simulink model "DriverInLoopSpeedgoat"  (R2021a)
settings: Solver=ode3  StartTime=0.0  StopTime=30  FixedStep=1e-3  RelTol=5e-3  EnableMultiTasking=on
StartFcn:
  | % tic
  | % tg2.start;
StopFcn:
  | % tg2.stop;
  | % toc
model workspace (MAT data in the model file):
  A_mu = 10
  B_reff = 8.386
  Cz = 7766.25
  DCT_Param.Transmission.Ratios = [3.78 2.18 1.43 1.03 0.935 0.84]
  DCT_Param.Transmission.Shaft_Inertia_Odd = 0.0023
  DCT_Param.Transmission.Shaft_Inertia_Even = 0.0009
  DCT_Param.Transmission.Shaft_Inertia_Output = 0.008
  DCT_Param.Transmission.Gear_Inertia = 0.001
  DCT_Param.Transmission.Gear_Efficiency = 0.94
  DCT_Param.Transmission.Gear_Ang_Vel_Thr = 0.01
  DCT_Param.Transmission.Shaft_Velocity_Odd = 0
  DCT_Param.Transmission.Shaft_Velocity_Even = 0
  DCT_Param.Transmission.Shaft_Velocity_Output = 0
  DCT_Param.Transmission.Gear_Initial_Velocity = 0
  DCT_Param.Transmission.Abstract.Compliance = 100000
  DCT_Param.Transmission.Abstract.Damping = 10000
  DCT_Param.Transmission.Abstract.Ratio_Time_Const = 0.05
  DCT_Param.Transmission.Abstract.Shift_Gear_Delay = 25
  DCT_Param.Clutch.Torque_Radius = 130
  DCT_Param.Clutch.Num_Friction_Surfaces = 4
  DCT_Param.Clutch.Engagement_Piston_Area = 0.001
  DCT_Param.Clutch.Kinetic_Friction_Coeff = 0.3
  DCT_Param.Clutch.Static_Friction_Coeff = 0.31
  DCT_Param.Clutch.Derating_Factor = 1
  DCT_Param.Clutch.Clutch_Velocity_Tolerance = 0.001
  DCT_Param.Clutch.Threshold_Pressure = 1
  DCT_Param.Clutch.Drag_Torque_Coeff = 0
  DCT_Param.Dog_Clutch.Max_Torque = 1000
  DCT_Param.Dog_Clutch.Teeth_Mean_Radius = 50
  DCT_Param.Dog_Clutch.Tooth_Height = 10
  DCT_Param.Dog_Clutch.Ring_Hub_Clearance = 3
  DCT_Param.Dog_Clutch.Ring_Stop_Stiffness = 1000000
  DCT_Param.Dog_Clutch.Ring_Stop_Damping = 1000
  DCT_Param.Dog_Clutch.Shift_Linkage_Damping = 100
  DCT_Param.Dog_Clutch.Max_Engage_Velocity = 1000000
  DCT_Param.Dog_Clutch.Tooth_Engage_Overlap = 3
  DCT_Param.Vehicle.Mass = 1600
  DCT_Param.Vehicle.Wheels_Per_Axle = 2
  DCT_Param.Vehicle.Distance_CG_FrontAxle = 1.7
  DCT_Param.Vehicle.Distance_CG_RearAxle = 2
  DCT_Param.Vehicle.Distance_CG_Ground = 0.5
  DCT_Param.Vehicle.Frontal_Area = 3
  DCT_Param.Vehicle.Aero_Drag_Coeff = 0.4
  DCT_Param.Vehicle.Initial_Velocity = 0
  DCT_Param.Vehicle.Final_Drive_Ratio = 3.7
  DCT_Param.Vehicle.Final_Drive_Efficiency = 0.86
  DCT_Param.Vehicle.Final_Drive_Vel_Thresh = 0.01
  DCT_Param.Vehicle.Side_Shaft_Inertia = 0.01
  DCT_Param.Vehicle.Side_Shaft_Initial_Velocity = 0
  DCT_Param.Vehicle.Tire.Radius = 0.312
  DCT_Param.Vehicle.Tire.Inertia = 0.5
  DCT_Param.Vehicle.Tire.Initial_Velocity = 0
  DCT_Param.Vehicle.Tire.Slip_Vel_Thresh = 0.1
  DCT_Param.Vehicle.Tire.Nominal_Vertical_Load = 4000
  DCT_Param.Vehicle.Tire.C_Coeff = 1.685
  DCT_Param.Vehicle.Tire.D_Coeff = [1.21 -0.037]
  DCT_Param.Vehicle.Tire.E_Coeff = [0.344 0.095 -0.02 0]
  DCT_Param.Vehicle.Tire.BCD_Coeff = [21.51 -0.163 0.245]
  DCT_Param.Vehicle.Tire.H_Coeff = [-0.002 0.002]
  DCT_Param.Vehicle.Tire.V_Coeff = [0 0]
  DCT_Param.ICE.Max_Power = 100000
  DCT_Param.ICE.Speed_At_Max_Power = 5500
  DCT_Param.ICE.Max_Speed = 7000
  DCT_Param.ICE.Stall_Speed = 200
  DCT_Param.ICE.Shaft_Inertia = 0.2
  DCT_Param.ICE.Initial_Velocity = 800
  DCT_Param.ICE.Idle_Ref_Spd = 800
  DCT_Param.ICE.Engine_Time_Constant = 0.2
  DCT_Param.ICE.Initial_Normalized_Throttle = 0
  DCT_Param.ICE.Speed_Threshold = 20
  DCT_Param.ICE.FC.Speed_Vector = [0 368.421052632 736.842105263 1105.26315789 1473.68421053 1842.10526316 2210.52631579 2578.94736842 2947.36842105 3315.78947368 3684.21052632 4052.63157895 4421.05263158 4789.47368421 5157.89473684 5526.31578947 5894.73684211 6263.15789474 6631.57894737 7000]
  DCT_Param.ICE.FC.Torque_Vector = [0 10.5263157895 21.0526315789 31.5789473684 42.1052631579 52.6315789474 63.1578947368 73.6842105263 84.2105263158 94.7368421053 105.263157895 115.789473684 126.315789474 136.842105263 147.368421053 157.894736842 168.421052632 178.947368421 189.473684211 200]
  DCT_Param.ICE.FC.Consumption_Table = [0.262945178015 0.225304787522 0.201465019624 0.191425874321 0.195187351614 0.212749451502 0.244112173984 0.289275519063 0.348239486736 0.421004077004 0.507569289868 0.607935125326 ... (400 elements, 20x20)]
  DCT_Param.Shift_Map_Example.Pedal_Positions = [0.1 0.4 0.5 0.9]
  DCT_Param.Shift_Map_Example.Upshift_Speeds = [11  20  26  34.5  43; 14  26  35  44.5  55; 17  31  42  52.5  65; 21  39  52  66.5  80]
  DCT_Param.Shift_Map_Example.Downshift_Speeds = [8.9  17  23.6  32.4  40.8; 11.5  22.7  32  41.6  52.2; 14  27  38.1  50  62; 18  33  48  62.6  76.2]
  DCT_Param.Shift_Map_ORIG.Pedal_Positions = [0.1 0.4 0.5 0.9]
  DCT_Param.Shift_Map_ORIG.Upshift_Speeds = [11.5  23.5  35.5  45.5  55.5; 14.5  26.5  38.5  48.5  58.5; 17.5  29.5  41.5  51.5  61.5; 20.5  32.5  44.5  54.5  64.5]
  DCT_Param.Shift_Map_ORIG.Downshift_Speeds = [8.5  20.5  32.5  42.5  52.5; 11.5  23.5  35.5  45.5  55.5; 14.5  26.5  38.5  48.5  58.5; 17.5  29.5  41.5  51.5  61.5]
  DCT_Param.Shift_Map_OPT.Pedal_Positions = [0.1 0.4 0.5 0.9]
  DCT_Param.Shift_Map_OPT.Upshift_Speeds = [17.8469  29.8469  35.8159  41.2981  46.3004; 19.2469  33.9778  43.9778  53.9778  63.9778; 24.5469  41.9778  62.1778  78.5778  106.9778; 27.5469  59.3778  99.0445  109.0445  119.0445]
  DCT_Param.Shift_Map_OPT.Downshift_Speeds = [14.8469  26.8469  32.8159  38.2981  43.3004; 16.2469  30.9778  40.9778  50.9778  60.9778; 21.5469  38.9778  59.1778  75.5778  103.9778; 24.5469  56.3778  96.0445  106.0445  116.0445]
  DCT_Param.Shift_Map.Pedal_Positions = [0.1 0.4 0.5 0.9]
  DCT_Param.Shift_Map.Upshift_Speeds = [11.5  23.5  35.5  45.5  55.5; 14.5  26.5  38.5  48.5  58.5; 17.5  29.5  41.5  51.5  61.5; 20.5  32.5  44.5  54.5  64.5]
  DCT_Param.Shift_Map.Downshift_Speeds = [8.5  20.5  32.5  42.5  52.5; 11.5  23.5  35.5  45.5  55.5; 14.5  26.5  38.5  48.5  58.5; 17.5  29.5  41.5  51.5  61.5]
  DCT_Param.Control.Clutch.Min_Lock_Pressure = 2000000
  DCT_Param.Control.Clutch.Max_Lock_Pressure = 5000000
  DCT_Param.Control.Clutch.Max_Unlock_Pressure = 500000
  DCT_Param.Control.Engine_Start_RPM = 800
  DCT_Param.Control.Engine_Stop_RPM = 790
  DCT_Param.Control.Mode_Logic_TS = 0.1
  DCT_Param.Control.ICE.Kp = 0.02
  DCT_Param.Control.ICE.Ki = 0.01
  DCT_Param.Control.Gen.Kp = 10
  DCT_Param.Control.Gen.Ki = 3
  DCT_Param.Control.Mot.Kp = 500
  DCT_Param.Control.Mot.Ki = 300
  DCT_Param.Control.Veh_Spd.Kp = 0.02
  DCT_Param.Control.Veh_Spd.Ki = 0.04
  DCT_Param.Driver.Kp = 400
  DCT_Param.Driver.Ki = 0.001
  DCT_Param.Driver.Pedal_Filter_Const = 0.01
  DCT_Param.Dog_Clutches.Pulse_Delay = 50
  DCT_Param.Dog_Clutches.Pulse_Length = 20
  DCT_Param.Animation.Teeth_Ratios = [0.338461538462 0.555555555556 0.916666666667 0.96 1.17948717949 1.92307692308]
  DCT_Param.Animation.Teeth_Ratios_Reverse = [0.458333333333 0.75]
  DCT_Param.Shift_Map_OPT506.Pedal_Positions = [0.1 0.4 0.5 0.9]
  DCT_Param.Shift_Map_OPT506.Upshift_Speeds = [18  30.2  48.3  67.3322  77.3429; 20.1  36.85  66.6178  76.7537  86.7537; 21.1  40.25  71.0189  81.0189  91.7873; 24.1  63.75  80.7523  105.9489  115.9489]
  DCT_Param.Shift_Map_OPT506.Downshift_Speeds = [15  27.2  45.3  64.3322  74.3429; 17.1  33.85  63.6178  73.7537  83.7537; 18.1  37.25  68.0189  78.0189  88.7873; 21.1  60.75  77.7523  102.9489  112.9489]
  DCT_Param.Shift_Map_OPTAbsRea176.Pedal_Positions = [0.1 0.4 0.5 0.9]
  DCT_Param.Shift_Map_OPTAbsRea176.Upshift_Speeds = [17.8469  29.8469  35.7875  44.0901  49.4243; 18.9219  34.1312  45.8256  59.7585  69.7585; 32.1719  43.4585  53.51  103.2151  114.6401; 35.1719  59.2585  99.5217  109.5217  119.5217]
  DCT_Param.Shift_Map_OPTAbsRea176.Downshift_Speeds = [14.8469  26.8469  32.7875  41.0901  46.4243; 15.9219  31.1312  42.8256  56.7585  66.7585; 29.1719  40.4585  50.51  100.2151  111.6401; 32.1719  56.2585  96.5217  106.5217  116.5217]
  DLC_XEnd = 236.9
  DLC_XStart = 175.9
  DLC_YStart = 3.2153
  D_reff = 0.25826
  Downshift_Speeds = [9.5625  23.0625  36.5625  47.8125; 12.9375  26.4375  39.9375  51.1875; 16.3125  29.8125  43.3125  54.5625; 19.6875  33.1875  46.6875  57.9375]
  EngRevLim = 7000
  Pedal_Positions = [0.1 0.4 0.5 0.9]
  SUS.Stiffness = 24000
  SUS.Damping.Constant = 1262
  SUS.Damping.Rebound = [4040 4950 2883 2043]
  SUS.Damping.Compression = [3600 3420 1863 1472]
  SUS.PistonSpeed = [0.05 0.1 0.3 0.6]
  SUS.UnsprungMass.Fr = 21.0693333333
  SUS.UnsprungMass.Rr = 21.0693333333
  Upshift_Speeds = [12.9375  26.4375  39.9375  51.1875; 16.3125  29.8125  43.3125  54.5625; 19.6875  33.1875  46.6875  57.9375; 33  52.5  77.25  100.5]
  VEH.Mass = 1181
  VEH.StaticNormalFrontLoad.FR = 264.666666667
  VEH.StaticNormalFrontLoad.FL = 264.666666667
  VEH.StaticNormalRearLoad.RR = 322
  VEH.StaticNormalRearLoad.RL = 322
  VEH.WheelBase = 3.075
  VEH.FrontAxlePositionfromCG = 1.515
  VEH.RearAxlePositionfromCG = 1.504
  VEH.HeightCG = 0.134
  VEH.FrontalArea = 2.11
  VEH.DragCoefficient = 0.33
  VEH.NumberOfWheelsPerAxle = 2
  VEH.Thread.FR = 1.705
  VEH.Thread.RR = 1.705
  VEH.PitchMomentInertia = 1922.66666667
  VEH.RollMomentInertia = 432.333333333
  VEH.YawMomentInertia = 2066
  VEH.SteeringRatio = 18
  VEH.TrackWidth = 1.922
  VEH.SprungMass = 1096.72266667
  VEH.InitialLongPosition = 0
  VEH.InitialLatPosition = 0
  VEH.InitialVertPosition = 0
  VEH.InitialRollAngle = 0
  VEH.InitialPitchAngle = 0
  VEH.InitialYawAngle = 0
  VEH.InitialLongVel = 0
  VEH.InitialLatVel = 0
  VEH.InitialVertVel = 0
  VEH.InitialRollRate = 0
  VEH.InitialPitchRate = 0
  VEH.InitialYawRate = 0
  V_o = 16.7
  V_xlow = 1
  WH.Tire.Radius.Front = 0.384
  WH.Tire.Radius.Rear = 0.401
  WH.Tire.Sidewall = 0.245
  WH.Tire.RollingResistCoeff = 0.0103
  WH.Tire.Magic.B = 10
  WH.Tire.Magic.C = 1.9
  WH.Tire.Magic.D = 1
  WH.Tire.Magic.E = 0.97
  WH.Tire.Magic.Bx = 12
  WH.Tire.Magic.Cx = 1.9
  WH.Tire.Magic.Dx = 0.72
  WH.Tire.Magic.Ex = 0.95
  WH.Tire.Magic.By = 12
  WH.Tire.Magic.Cy = 1.3
  WH.Tire.Magic.Dy = 0.75
  WH.Tire.Magic.Ey = 0.2
  WH.Tire.Front.Ky = 40000
  WH.Tire.Rear.Ky = 40000
  WH.Tire.Kz = 320000
  WH.Tire.Damping = 100
  WH.Inertia = 1.00333333333
  WH.Mass = 11.4333333333
  WH.DampingCoefficient = 0.01
  WH.VelocityTol = 0.1
  a = 1.4
  alpha_max = 1.5
  alpha_min = -1.5
  b = 1.8
  c_zo = 209651
  epsilon = 0.1
  h = 0.134
  path.ISO3888p2.x = [0 2 12 25.5 36.5 49 61]
  path.ISO3888p2.y = [0 0 0 3.725 3.725 0 0]
  path.ISO3888p2.ylb = [1.225 1.225 1.225 4.725 4.725 1.5 1.5]
  path.ISO3888p2.yrb = [-1.225 -1.225 -1.225 2.225 2.225 -1.5 -1.5]
  path.CUSC.x = [10.668 21.336 36.576 54.864 73.152]
  path.CUSC.y = [0 0 5.1816 0 0]
  path.CUSC.ylb = [1.2192 1.2192 7.0104 1.8288 1.8288]
  path.CUSC.yrb = [-1.2192 -1.2192 3.3528 -1.8288 -1.8288]
  pio = 220000
  q_Fcx = 0
  q_Fz2 = 15.4
  q_Fzy = 0
  q_reo = 0.9974
  q_sx1 = -0.007764
  q_sx10 = 0.2824
  q_sx11 = 5.349
  q_sx12 = 0
  q_sx13 = 0
  q_sx14 = 0
  q_sx2 = 1.1915
  q_sx3 = 0.013948
  q_sx4 = 4.912
  q_sx5 = 1.02
  q_sx6 = 22.83
  q_sx7 = 0.7104
  q_sx8 = -0.023393
  q_sx9 = 0.6581
  q_sy1 = 0.00702
  q_sy2 = 0
  q_sy3 = 0.001515
  q_sy4 = 8.514e-05
  q_sy5 = 0
  q_sy6 = 0
  q_sy7 = 0.9008
  q_sy8 = -0.4089
  q_v1 = 0.0007742
  q_v2 = 0.04667
  r_Bx1 = 12.531
  r_Bx2 = 9.532
  r_Bx3 = 0
  r_By1 = 10.615
  r_By2 = 7.705
  r_By3 = 3.433e-06
  r_By4 = 0
  r_Cx1 = 1.019
  r_Cy1 = 1.0585
  r_Ex1 = -0.4487
  r_Ex2 = -0.4726
  r_Ey1 = 0.3132
  r_Ey2 = 7.63e-06
  r_Hx1 = 0.0002374
  r_Hy1 = 0.011646
  r_Hy2 = 7.63e-06
  r_Vy1 = 0.05654
  r_Vy2 = 7.63e-06
  r_Vy3 = 0
  r_Vy4 = 99.9
  r_Vy5 = 2
  r_Vy6 = 15.814
  r_o = 0.3135
  vehWidth = 2
  w = 1
  xdot_ref = 13.4112
values from neighbouring files (symbols this model uses):
  stop_pedal = 20    [config_test.m]
undefined symbols (not defined in the file or in its folder): ESP_mode
libraries: autolibutils x7, simulink x6, slrealtimeutilitieslib x2, slrealtimeiplib x2, sim3dlib x1, sim3dautolib x1, pid_lib x1, slrealtimeobsoletelib x1, dspstat3 x1
(part 1 of 2)
settings Model: SimulationMode=accelerator  Creator=The MathWorks, Inc.  LastModifiedBy=indeevar
settings SolverCC: ConcurrentTasks=on  ZeroCrossAlgorithm=Adaptive  AlgebraicLoopSolver=TrustRegion  PositivePriorityOrder=on  AutoInsertRateTranBlk=on  InsertRTBMode=Never (minimum delay)  DecoupledContinuousIntegration=on  MinimalZcImpactIntegration=on
settings DataIOCC: SaveFormat=StructureWithTime
settings OptimizationCC: BlockReduction=off  OptimizeBlockIOStorage=off  BufferReuse=off  GlobalBufferReuse=off  ExpressionFolding=off  LocalBlockOutputs=off  ZeroExternalMemoryAtStartup=off  ZeroInternalMemoryAtStartup=off  OptimizeDataStoreBuffers=off  BusAssignmentInplaceUpdate=off
settings DebuggingCC: SignalInfNanChecking=error  ArtificialAlgebraicLoopMsg=none  IgnoredZcDiagnostic=none  InheritedTsInSrcMsg=none  TasksWithSamePriorityMsg=none  SigSpecEnsureSampleTimeMsg=none  ModelReferenceSymbolNameMessage=none  ModelReferenceExtraNoncontSigs=none  SFMachineParentedDataDiag=warning  ArithmeticOperatorsInVariantConditions=warning
settings ModelReferenceCC: UpdateModelReferenceTargets=IfOutOfDate  ModelReferenceMinAlgLoopOccurrences=on  PropagateSignalLabelsOutOfModel=off
settings SFSimCC: SimUseLocalCustomCode=off  CustomCodeUndefinedFunction=UseInterfaceOnly
settings RTWCC: Description=Generic Real-Time Target  RTWUseLocalCustomCode=off  Toolchain=Simulink Real-Time Toolchain  BuildConfiguration=Faster Runs  TargetLang=C++  RTWCompilerOptimization=on
settings CodeAppCC: MaxIdLength=95
settings GRTTargetCC: TargetLangStandard=C++03 (ISO)  CodeInterfacePackaging=C++ class

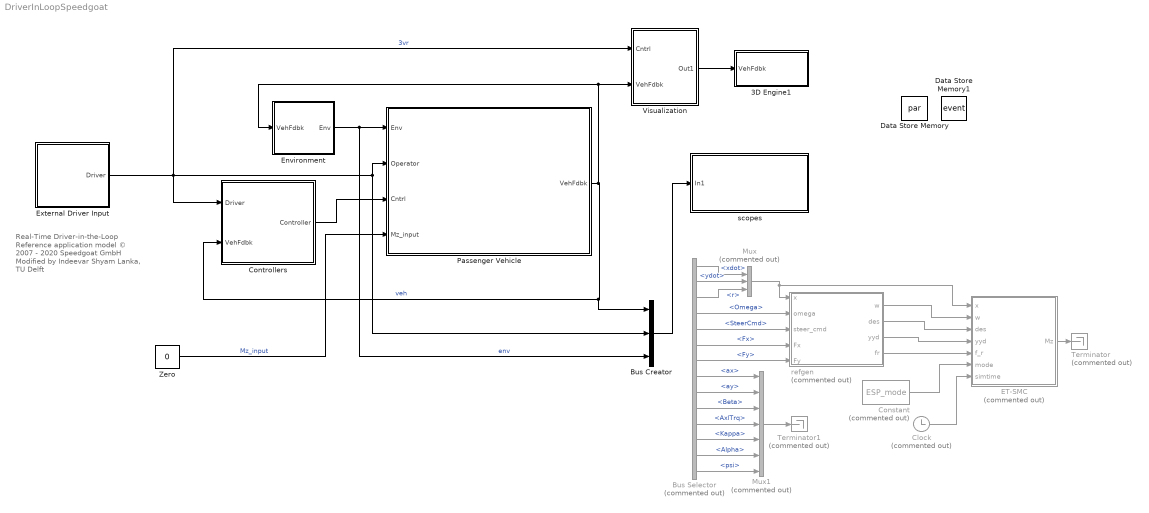
== system DriverInLoopSpeedgoat ==
  note: Real-Time Driver-in-the-Loop
      |
      | Reference application model
      | © 2007 - 2020 Speedgoat GmbH
      |
      | Modified by
      | Indeevar Shyam Lanka, TU Delft
  3D Engine1 : Subsystem  Variant=on  VariantControlMode=label  LabelModeActiveChoice=0  mask(3D Engine){engine3D=Disabled, SceneDesc=Open surface, dt3D=0.02, defaultPos=User-specified, X_o=0, Y_o=0, Z_o=0, phi_o=0, theta_o=0, psi_o=0}
      mask prompts: engine3D "3D Engine"; SceneDesc "Scene:"; dt3D "Engine frame rate, dt3D [s]:"; X_o "Initial longitudinal position, X_o [m]:"; Y_o "Initial lateral position, Y_o [m]:"; Z_o "Initial vertical position, Z_o [m]:"; phi_o "Initial roll angle, phi_o [rad]:"; theta_o "Initial pitch angle, theta_o [rad]:"; psi_o "Initial yaw angle, psi_o [rad]:"
      mask help: This subsystem contains the interface blocks which permit the display of the vehicle in the 3D virtual environment. Enable it to view the simulation progress, disable it to inhibit the display.
      mask init:
      | switch get_param(gcb,'engine3D')
      |     case 'Disabled'
      |         set_param(gcb,'OverrideUsingVariant','0')
      |         try
      |             set_param([bdroot '/Environment/Ground Feedback'],'OverrideUsingVariant','0')
      |         catch
      |             disp('Warning: No ground feedback sensor not set')
      |         end
      |     case 'Enabled'
      |         set_param(gcb,'OverrideUsingVariant','1')
      |         try
      |             set_param([bdroot '/Environment/Ground Feedback'],'OverrideUsingVariant','1')
      |         catch
      |             disp('Warning: No ground feedback sensor not set')
      |         end
      |     otherwise
      |         set_param(gcb,'OverrideUsingVariant','0')
      | end
      settings: AttributesFormatString=|
      | %<SceneDesc>
      | %<engine3D>
      mask Help: eval('vdynblkshelp(''vdynblks3dengine'')');
      mask TypeOptions engine3D: Enabled | Disabled
      mask Callback engine3D:
      | switch get_param(gcb,'engine3D')
      |     case 'Disabled'
      |         set_param(gcb,'OverrideUsingVariant','0')
      |     case 'Enabled'
      |        set_param(gcb,'OverrideUsingVariant','1')
      |     otherwise
      |        set_param(gcb,'OverrideUsingVariant','0')
      | end
      mask TypeOptions SceneDesc: 3D Engine/Simulation 3D Scene Configuration/SceneDesc
      mask Callback SceneDesc:
      | defaultStatus = get_param(gcb,'defaultPos');
      | if strcmp(defaultStatus,'Recommended for scene')
      | sceneType = get_param(gcb,'SceneDesc');
      | switch sceneType
      |     case 'Straight road'
      |         set_param(gcb,'X_o', '-118')
      |         set_param(gcb,'Y_o', '3.125')
      |         set_param(gcb,'Z_o', '0')
      |         set_param(gcb,'phi_o', '0')
      |         set_param(gcb,'theta_o', '0')
      |         set_param(gcb,'psi_o', '0')
      |     case 'Curved road'
      |         set_param(gcb,'X_o', '0.2')
      |         set_param(gcb,'Y_o', '-1605.0')
      |         set_param(gcb,'Z_o', '0')
      |         set_param(gcb,'phi_o', '0')
      |         set_param(gcb,'theta_o', '0')
      |         set_param(gcb,'psi_o', '-156*pi/180')
      |     case 'Parking lot'
      |         set_param(gcb,'X_o', '-104.0')
      |         set_param(gcb,'Y_o', '-9.7')
      |         set_param(gcb,'Z_o', '0')
      |         set_param(gcb,'phi_o', '0')
      |         set_param(gcb,'theta_o', '0')
      |         set_param(gcb,'psi_o', '0')
      |     case 'Double lane change'
      |         set_param(gcb,'X_o', '0')
      |         set_param(gcb,'Y_o', '3.125')
      |         set_param(gcb,'Z_o', '0')
      |         set_param(gcb,'phi_o', '0')
      |         set_param(gcb,'theta_o', '0')
      |         set_param(gcb,'psi_o', '0')
      |     case 'Open surface'
      |         set_param(gcb,'X_o', '0')
      |         set_param(gcb,'Y_o', '0')
      |         set_param(gcb,'Z_o', '0')
      |         set_param(gcb,'phi_o', '0')
      |         set_param(gcb,'theta_o', '0')
      |         set_param(gcb,'psi_o', '0')
      |     case 'US highway'
      |         set_param(gcb,'X_o', '3592.00')
      |         set_param(gcb,'Y_o', '2617.00')
      |         set_param(gcb,'Z_o', '-1.0')
      |         set_param(gcb,'phi_o', '0')
      |         set_param(gcb,'theta_o', '0')
      |         set_param(gcb,'psi_o', '0')
      |     case 'US city block'
      |         set_param(gcb,'X_o', '-125.19')
      |         set_param(gcb,'Y_o', '1.65')
      |         set_param(gcb,'Z_o', '-0.04')
      |         set_param(gcb,'phi_o', '0')
      |         set_param(gcb,'theta_o', '0')
      |         set_param(gcb,'psi_o', '0')
      |     case 'Large parking lot'
      |         set_param(gcb,'X_o', '45.0')
      |         set_param(gcb,'Y_o', '54.7')
      |         set_param(gcb,'Z_o', '0.0')
      |         set_param(gcb,'phi_o', '0')
      |         set_param(gcb,'theta_o', '0')
      |         set_param(gcb,'psi_o', '-pi/2')
      |     case 'Virtual Mcity'
      |         set_param(gcb,'X_o', '-26.0')
      |         set_param(gcb,'Y_o', '76.0')
      |         set_param(gcb,'Z_o', '0.0')
      |         set_param(gcb,'phi_o', '0')
      |         set_param(gcb,'theta_o', '0')
      |         set_param(gcb,'psi_o', '-40*pi/180')
      |     otherwise
      |         set_param(gcb,'X_o', '0')
      |         set_param(gcb,'Y_o', '0')
      |         set_param(gcb,'Z_o', '0')
      |         set_param(gcb,'phi_o', '0')
      |         set_param(gcb,'theta_o', '0')
      |         set_param(gcb,'psi_o', '0')
      | end
      | end
      mask TypeOptions defaultPos: Recommended for scene | User-specified
      mask DialogControl engineConfig Prompt: 3D Engine Settings
      mask DialogControl posSetup Prompt: Initial vehicle position
      mask DialogControl posSetupDesc Prompt: To use these initial vehicle positions, first Apply the initial values and then click Update the model workspaces with the initial values.
      mask DialogControl setModelPos Prompt: Update model workspaces with initial values
      mask DialogControl setModelPos Callback:
      | if strcmp(get_param(bdroot(gcb),'SimulationStatus'),'stopped')
      |     sceneType = get_param(gcb,'SceneDesc');
      |     rootModel = bdroot(gcb);
      |     ws = get_param(rootModel, 'modelworkspace');
      |     VEH = getVariable(ws,'VEH');
      |     ParamList={'X_o',[1,1],{};'Y_o',[1,1],{};'Z_o',[1,1],{};'phi_o',[1,1],{'gte',-pi/2;'lte',pi/2};'theta_o',[1,1],{'gte',-pi/2;'lte',pi/2};'psi_o',[1,1],{'gte',-2*pi;'lte',2*pi}};
      |     paramStruct = autoblkscheckparams(gcb, '3D Engine',ParamList);
      |     VEH.InitialLongPosition = paramStruct.X_o;
      |     VEH.InitialLatPosition = paramStruct.Y_o;
      |     VEH.InitialVertPosition = paramStruct.Z_o;
      |     VEH.InitialRollAngle = paramStruct.phi_o;
      |     VEH.InitialPitchAngle = paramStruct.theta_o;
      |     VEH.InitialYawAngle = paramStruct.psi_o;
      |     assignin(ws,'VEH',VEH);
      |     modelList = {'PassVeh14DOF','PassVeh7DOF'};
      |     for idx =1:length(modelList)
      | %         try
      |             load_system(modelList{idx});
      |             ws = get_param(modelList{idx}, 'modelworkspace');
      |             assignin(ws,'VEH',VEH);
      |             save_system(modelList{idx});
      |             close_system(modelList{idx});
      | %         catch
      | %             disp(['Cannot find ' modelList{idx}])
      | %         end
      |     end
      | end
      mask Display: disp('3D Engine')
  Bus Creator : BusCreator  Inputs=3
  Bus Selector : BusSelector  Commented=on  OutputSignals=veh.Body.xdot,veh.Body.ydot,veh.Body.r,veh.Wheels.Omega,3vr.SteerCmd,veh.Wheels.Fx,veh.Wheels.Fy,veh.Body.ax,veh.Body.ay,veh.Body.Beta,veh.Driveline.AxlTrq,veh.Wheels.Kappa,veh.Wheels.Alpha,veh.Body.psi
  Clock : Clock  Commented=on
  Constant : Constant  Commented=on  Value=ESP_mode
  Controllers : Subsystem
      mask Display: image('SystemControllers.png')
  Data Store Memory : DataStoreMemory  DataStoreName=par  ReadBeforeWriteMsg=warning  WriteAfterWriteMsg=warning  WriteAfterReadMsg=warning  InitialValue=[0,0,0,0,0,0,0,0,0,0,0,0,0]  ShowAdditionalParam=off
  Data Store Memory1 : DataStoreMemory  DataStoreName=event  ReadBeforeWriteMsg=warning  WriteAfterWriteMsg=warning  WriteAfterReadMsg=warning  InitialValue=zeros(13,1)  ShowAdditionalParam=off
  ET-SMC : MATLAB Function  Commented=on  TreatAsAtomicUnit=on
  Environment : Subsystem
      mask Display: disp('Environment')
  External Driver Input : Subsystem  Variant=on  VariantControlMode=label  LabelModeActiveChoice=G29 connected to Host
      mask Display: image('driverlatlong.png');
  Mux : Mux  Commented=on  Inputs=3
  Mux1 : Mux  Commented=on  Inputs=7
  Passenger Vehicle : Subsystem
      mask Display: image('PassengerVehicle.png')
  Terminator : Terminator  Commented=on
  Terminator1 : Terminator  Commented=on
  Visualization : Subsystem
      mask Display: disp('Visualization')
  Zero : Constant  Value=0  OutDataTypeStr=Inherit: Inherit via back propagation
  refgen : MATLAB Function  Commented=on  TreatAsAtomicUnit=on
  scopes : Subsystem
  wires:
  Passenger Vehicle/1(VehFdbk) -> Visualization/2(VehFdbk), Environment/1(VehFdbk), Bus Creator/1, Controllers/2(VehFdbk)  "veh"
  Controllers/1(Controller) -> Passenger Vehicle/3(Cntrl)
  Environment/1(Env) -> Passenger Vehicle/1(Env), Bus Creator/3  "env"
  External Driver Input/1(Driver) -> Visualization/1(Cntrl), Bus Creator/2, Passenger Vehicle/2(Operator), Controllers/1(Driver)  "3vr"
  Zero/1 -> Passenger Vehicle/4(Mz_input)  "Mz_input"
  Visualization/1(Out1) -> 3D Engine1/1(VehFdbk)
  Bus Creator/1 -> scopes/1(In1)
  Bus Selector/1 -> Mux/1  "<xdot>"
  ET-SMC/1(Mz) -> Terminator/1
  Bus Selector/2 -> Mux/2  "<ydot>"
  Bus Selector/3 -> Mux/3  "<r>"
  Bus Selector/6 -> refgen/4(Fx)  "<Fx>"
  Bus Selector/7 -> refgen/5(Fy)  "<Fy>"
  Bus Selector/4 -> refgen/2(omega)  "<Omega>"
  refgen/2(des) -> ET-SMC/3(des)
  refgen/3(yyd) -> ET-SMC/4(yyd)
  refgen/4(fr) -> ET-SMC/5(f_r)
  Bus Selector/8 -> Mux1/1  "<ax>"
  Bus Selector/5 -> refgen/3(steer_cmd)  "<SteerCmd>"
  Bus Selector/9 -> Mux1/2  "<ay>"
  Bus Selector/10 -> Mux1/3  "<Beta>"
  Bus Selector/11 -> Mux1/4  "<AxlTrq>"
  Bus Selector/12 -> Mux1/5  "<Kappa>"
  Bus Selector/13 -> Mux1/6  "<Alpha>"
  Bus Selector/14 -> Mux1/7  "<psi>"
  Mux1/1 -> Terminator1/1
  refgen/1(w) -> ET-SMC/2(w)
  Mux/1 -> refgen/1(x), ET-SMC/1(x)
  Constant/1 -> ET-SMC/6(mode)
  Clock/1 -> ET-SMC/7(simtime)

== system DriverInLoopSpeedgoat/3D Engine1 ==
  note: 1) Add Subsystem or Model blocks as valid variant choices.
      | 2) You cannot connect blocks at this level. At simulation, connectivity is automatically
      | determined, based on the active variant and port name matching.
  VehFdbk : Inport
  3D Engine : Subsystem  VariantControl=1
  3D Engine Disabled : Subsystem  VariantControl=0

== system DriverInLoopSpeedgoat/Controllers ==
  Driver : Inport
  VehFdbk : Inport  Port=2
  Brake Controller : Subsystem
  Bus Creator : BusCreator  Inputs=1
  Bus Creator1 : BusCreator  Inputs=1
  Bus Creator2 : BusCreator  Inputs=1
  Bus Creator3 : BusCreator  Inputs=3
  Bus Selector : BusSelector  OutputSignals=Body.xdot,Wheels.Kappa
  Bus Selector1 : BusSelector  OutputSignals=Driveline.EngSpd,Driveline.PropShftSpd
  Bus Selector2 : BusSelector  OutputSignals=Accel,ShiftUp,ShiftDn,ToggleMode,Brake
  ECU : Subsystem
  Man_speed_control : Subsystem
  Transmission Controller : Subsystem
  Controller : Outport  VectorParamsAs1DForOutWhenUnconnected=off
  tag scope: GearCmdVis=global
  wires:
  Brake Controller/1(PCmd) -> Bus Creator2/1  "PrsCmd"
  Bus Creator3/1 -> Controller/1  "Controller"
  Bus Creator2/1 -> Bus Creator3/3  "Brake"
  Bus Creator/1 -> Bus Creator3/1  "ECU"
  Driver/1 -> Bus Selector2/1
  Transmission Controller/1(Gear) -> Bus Creator1/1, [GearCmdVis]  "GearCmd"
  Bus Selector1/2 -> Transmission Controller/6(PrpSpd)  "<PropShftSpd>"
  Bus Selector2/5 -> Brake Controller/1(BrkCmd)  "<Brake>"
  VehFdbk/1 -> Bus Selector1/1, Bus Selector/1
  Bus Selector/1 -> Brake Controller/2(xdot), Man_speed_control/1(u)  "<xdot>"
  Bus Selector2/1 -> Man_speed_control/2(Init_acc)  "<Accel>"
  Bus Selector/2 -> Brake Controller/3(kappa)  "<Kappa>"
  ECU/1(Trq Cmd1) -> Bus Creator/1  "EngTrqCmd"
  Bus Creator1/1 -> Bus Creator3/2  "Transmission"
  Bus Selector1/1 -> Transmission Controller/5(EngSpd), ECU/2(EngSpd)  "<EngSpd>"
  Bus Selector2/2 -> Transmission Controller/2(UpReq)  "<ShiftUp>"
  Bus Selector2/3 -> Transmission Controller/3(DownReq)  "<ShiftDn>"
  Bus Selector2/4 -> Transmission Controller/4(ToggleMode)  "<ToggleMode>"
  Man_speed_control/1(<Accel>) -> Transmission Controller/1(Accel), ECU/1(<Accel>)

== system DriverInLoopSpeedgoat/Environment ==
  VehFdbk : Inport
  Bus Creator1 : BusCreator  Inputs=2
  Bus Creator3 : BusCreator  Inputs=2
  Constant3 : Constant  Value=0
  Constant4 : Constant  Value=0
  Constant5 : Constant  Value=0
  Friction Scaling : Subsystem  Variant=on  VariantControlMode=label  LabelModeActiveChoice=0
  Ground Height : Subsystem  Variant=on  VariantControlMode=label  LabelModeActiveChoice=0
  Vector Concatenate : Concatenate  NumInputs=3
  Env : Outport  VectorParamsAs1DForOutWhenUnconnected=off
  wires:
  Friction Scaling/1(mu) -> Bus Creator3/2  "mu"
  Constant5/1 -> Vector Concatenate/3  "Z"
  Vector Concatenate/1 -> Bus Creator1/1  "Wind"
  Constant3/1 -> Vector Concatenate/1  "X"
  Constant4/1 -> Vector Concatenate/2  "Y"
  Bus Creator3/1 -> Bus Creator1/2  "Gnd"
  Bus Creator1/1 -> Env/1
  VehFdbk/1 -> Friction Scaling/1(VehFdbk)
  Ground Height/1(z) -> Bus Creator3/1

== system DriverInLoopSpeedgoat/External Driver Input ==
  note: 1) Add Subsystem or Model blocks as valid variant choices.
      | 2) You cannot connect blocks at this level. At simulation, connectivity is automatically
      | determined, based on the active variant and port name matching.
  External Driver - Host : Subsystem  VariantControl=G29 connected to Host
      mask Display: image('driverlatlong.png');
  External Driver - Speedgoat : Subsystem  TreatAsAtomicUnit=on  VariantControl=G20 connected to Speedgoat  mask{selection=LogitechG920}
      mask prompts: selection "Select External Steering Device:"
      settings: MinAlgLoopOccurrences=on
      mask TypeOptions selection: LogitechG920 | LogitechF310 | ThrustmasterT150 | FanatecClubSport
      mask Callback selection:
      | % set variant for Axes mapping
      | set_param([gcb, '/MapAndScaleAxes'],...
      |           'OverrideUsingVariant', get_param(gcb, 'selection'));
      | 
      | % set variant for Button mapping
      | set_param([gcb, '/MapButtons'],...
      |           'OverrideUsingVariant', get_param(gcb, 'selection'));
      mask Display: image('driverlatlong.png');
  Driver : Outport

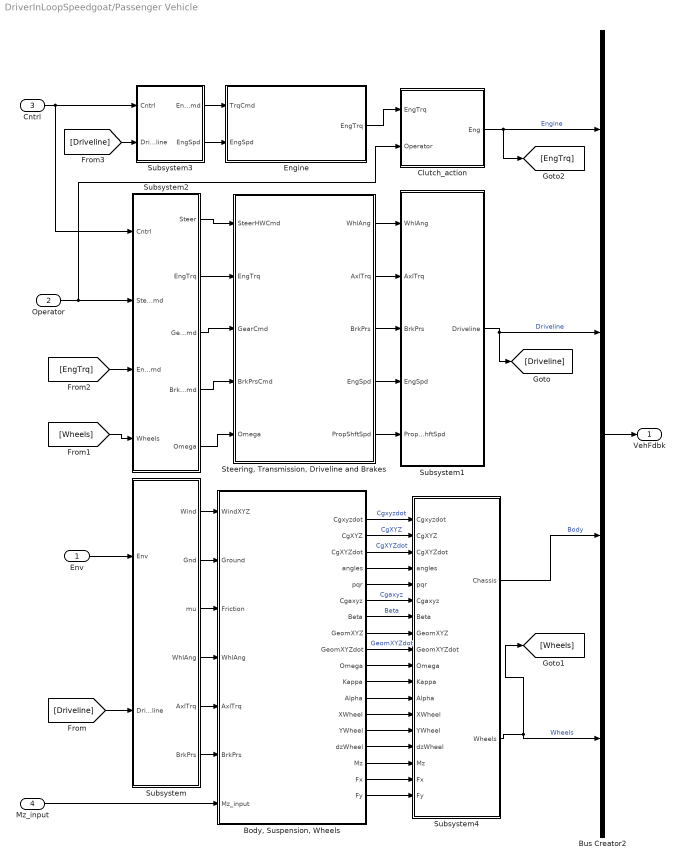
== system DriverInLoopSpeedgoat/Passenger Vehicle ==
  Env : Inport
  Operator : Inport  Port=2
  Cntrl : Inport  Port=3
  Mz_input : Inport  Port=4
  "Body, Suspension, Wheels" : Subsystem  Variant=on  VariantControlMode=label  LabelModeActiveChoice=3
  Bus Creator2 : BusCreator  Inputs=4
  Clutch_action : Subsystem
  Engine : Subsystem  Variant=on  VariantControlMode=label  LabelModeActiveChoice=0
  "Steering, Transmission, Driveline and Brakes" : Subsystem  Variant=on  VariantControlMode=label  LabelModeActiveChoice=0
  Subsystem : Subsystem
  Subsystem1 : Subsystem
  Subsystem2 : Subsystem
  Subsystem3 : Subsystem
  Subsystem4 : Subsystem
  VehFdbk : Outport  VectorParamsAs1DForOutWhenUnconnected=off
  wires:
  "Body, Suspension, Wheels"/9(GeomXYZdot) -> Subsystem4/9(GeomXYZdot)  "GeomXYZdot"
  "Body, Suspension, Wheels"/11(Kappa) -> Subsystem4/11(Kappa)
  Subsystem4/2(Wheels) -> Bus Creator2/4, [Wheels]  "Wheels"
  Subsystem/1(Wind) -> "Body, Suspension, Wheels"/1(WindXYZ)
  Engine/1(EngTrq) -> Clutch_action/1("EngTrq ")
  Subsystem2/2(EngTrq) -> "Steering, Transmission, Driveline and Brakes"/2(EngTrq)
  "Body, Suspension, Wheels"/12(Alpha) -> Subsystem4/12(Alpha)
  Env/1 -> Subsystem/1(Env)
  "Steering, Transmission, Driveline and Brakes"/3(BrkPrs) -> Subsystem1/3(BrkPrs)
  "Body, Suspension, Wheels"/14(YWheel) -> Subsystem4/14(YWheel)
  "Body, Suspension, Wheels"/1(Cgxyzdot) -> Subsystem4/1(Cgxyzdot)  "Cgxyzdot"
  "Body, Suspension, Wheels"/13(XWheel) -> Subsystem4/13(XWheel)
  Cntrl/1 -> Subsystem3/1(Cntrl), Subsystem2/1(Cntrl)
  "Body, Suspension, Wheels"/2(CgXYZ) -> Subsystem4/2(CgXYZ)  "CgXYZ"
  "Body, Suspension, Wheels"/7(Beta) -> Subsystem4/7(Beta)  "Beta"
  "Body, Suspension, Wheels"/6(Cgaxyz) -> Subsystem4/6(Cgaxyz)  "Cgaxyz"
  "Steering, Transmission, Driveline and Brakes"/4(EngSpd) -> Subsystem1/4(EngSpd)
  "Body, Suspension, Wheels"/8(GeomXYZ) -> Subsystem4/8(GeomXYZ)
  Subsystem3/1(EngTrqCmd) -> Engine/1(TrqCmd)
  Subsystem/2(Gnd) -> "Body, Suspension, Wheels"/2(Ground)
  Clutch_action/1(Eng) -> [EngTrq], Bus Creator2/1  "Engine"
  [Driveline] -> Subsystem3/2(Driveline)
  [EngTrq] -> Subsystem2/3(EngTrqCmd)
  Bus Creator2/1 -> VehFdbk/1
  Subsystem2/4(BrkPrsCmd) -> "Steering, Transmission, Driveline and Brakes"/4(BrkPrsCmd)
  Subsystem2/5(Omega) -> "Steering, Transmission, Driveline and Brakes"/5(Omega)
  "Body, Suspension, Wheels"/3(CgXYZdot) -> Subsystem4/3(CgXYZdot)  "CgXYZdot"
  "Body, Suspension, Wheels"/15(dzWheel) -> Subsystem4/15(dzWheel)
  [Driveline] -> Subsystem/2(Driveline)
  Operator/1 -> Clutch_action/2(Operator), Subsystem2/2(SteerCmd)
  [Wheels] -> Subsystem2/4(Wheels)
  Subsystem/5(AxlTrq) -> "Body, Suspension, Wheels"/5(AxlTrq)
  Subsystem1/1(Driveline) -> [Driveline], Bus Creator2/2  "Driveline"
  "Steering, Transmission, Driveline and Brakes"/2(AxlTrq) -> Subsystem1/2(AxlTrq)
  "Body, Suspension, Wheels"/4(angles) -> Subsystem4/4(angles)
  "Steering, Transmission, Driveline and Brakes"/5(PropShftSpd) -> Subsystem1/5(PropShftSpd)
  Subsystem/4(WhlAng) -> "Body, Suspension, Wheels"/4(WhlAng)
  Subsystem2/1(Steer) -> "Steering, Transmission, Driveline and Brakes"/1(SteerHWCmd)
  "Body, Suspension, Wheels"/5(pqr) -> Subsystem4/5(pqr)
  Subsystem3/2(EngSpd) -> Engine/2(EngSpd)
  "Steering, Transmission, Driveline and Brakes"/1(WhlAng) -> Subsystem1/1(WhlAng)
  Subsystem/6(BrkPrs) -> "Body, Suspension, Wheels"/6(BrkPrs)
  Subsystem2/3(GearCmd) -> "Steering, Transmission, Driveline and Brakes"/3(GearCmd)
  Subsystem/3(mu) -> "Body, Suspension, Wheels"/3(Friction)
  "Body, Suspension, Wheels"/10(Omega) -> Subsystem4/10(Omega)
  Subsystem4/1(Chassis) -> Bus Creator2/3  "Body"
  "Body, Suspension, Wheels"/16(Mz) -> Subsystem4/16(Mz)
  Mz_input/1 -> "Body, Suspension, Wheels"/7(Mz_input)
  "Body, Suspension, Wheels"/17(Fx) -> Subsystem4/17(Fx)
  "Body, Suspension, Wheels"/18(Fy) -> Subsystem4/18(Fy)

== system DriverInLoopSpeedgoat/Visualization ==
  note: Vehicle Response
  note: Driver Commands
  Cntrl : Inport
  VehFdbk : Inport  Port=2
  Acceleration Cmd : LinearGaugeBlock  ScaleMax=1
  Brake Cmd : LinearGaugeBlock  ScaleMax=1
  Engine Tach [rpm] : CircularGaugeBlock  ScaleMax=8000  TickInterval=1000
  Handwheel Angle [deg] : SemiCircularGaugeBlock  ScaleMin=-300  ScaleMax=300  TickInterval=60
  Lateral Acceleration [g] : SemiCircularGaugeBlock  ScaleMin=-1  ScaleMax=1  TickInterval=0.5
  Select_signals : Subsystem
  Speed [mph] : CircularGaugeBlock
  Out1 : Outport
  wires:
  Cntrl/1 -> Select_signals/1(Cntrl)
  VehFdbk/1 -> Select_signals/2(VehFdbk)  "VehFdbk"
  Select_signals/1(3DEngine) -> Out1/1

== system DriverInLoopSpeedgoat/scopes ==
  In1 : Inport
  Bus Selector : BusSelector  OutputSignals=veh.Body.xdot,veh.Body.ydot,veh.Body.r,veh.Body.ax,veh.Body.ay,veh.Body.Y,veh.Body.GeomY,veh.Driveline.AxlTrq,veh.Wheels.Kappa,veh.Wheels.Alpha,veh.Wheels.Fx,veh.Wheels.Fy
  Scope : Scope  NumInputPorts=5
  Scope1 : Scope  NumInputPorts=5
  Terminator1 : Terminator
  Terminator2 : Terminator
  wires:
  Bus Selector/4 -> Terminator2/1  "<ax>"
  Bus Selector/10 -> Scope1/3  "<Alpha>"
  Bus Selector/1 -> Terminator1/1  "<xdot>"
  Bus Selector/3 -> Scope/5  "<r>"
  Bus Selector/2 -> Scope/3  "<ydot>"
  Bus Selector/6 -> Scope/1  "<Y>"
  Bus Selector/5 -> Scope/4  "<ay>"
  In1/1 -> Bus Selector/1
  Bus Selector/7 -> Scope/2  "<GeomY>"
  Bus Selector/8 -> Scope1/1  "<AxlTrq>"
  Bus Selector/11 -> Scope1/4  "<Fx>"
  Bus Selector/12 -> Scope1/5  "<Fy>"
  Bus Selector/9 -> Scope1/2  "<Kappa>"

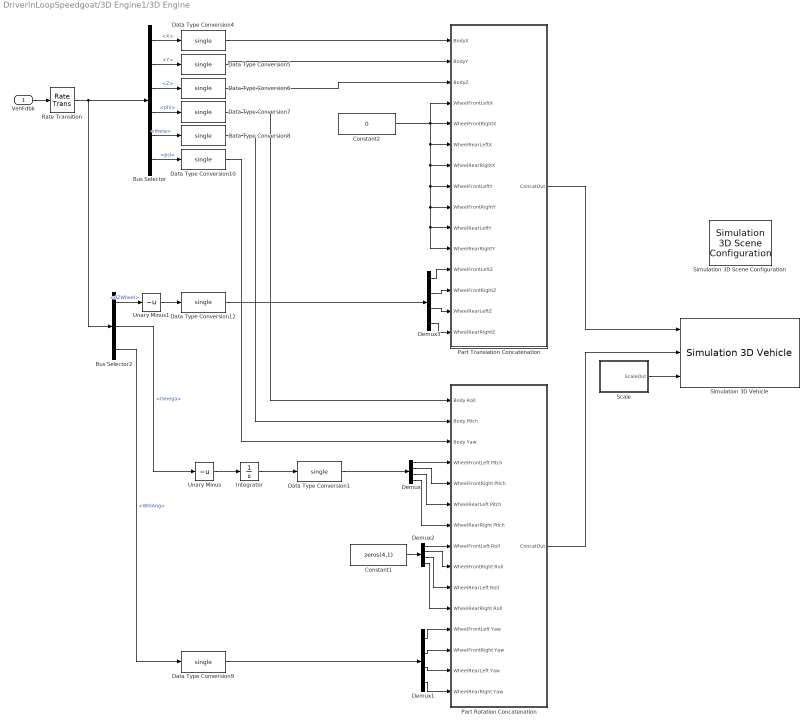
== system DriverInLoopSpeedgoat/3D Engine1/3D Engine ==
  VehFdbk : Inport
  Bus Selector : BusSelector  OutputSignals=X,Y,Z,phi,theta,psi
  Bus Selector2 : BusSelector  OutputSignals=dZWheel,Omega,WhlAng
  Constant1 : Constant  Value=zeros(4,1)  OutDataTypeStr=single
  Constant2 : Constant  Value=0  OutDataTypeStr=single
  Data Type Conversion{1,4..10,12} (9 alike) : DataTypeConversion  OutDataTypeStr=single
  Demux{,1..3} (4 alike) : Demux
  Integrator : Integrator  WrapState=on  WrappedStateUpperValue=2*pi  WrappedStateLowerValue=0  ZeroCross=off
  Part Rotation Concatenation : Subsystem
  Part Translation Concatenation : Subsystem
  Rate Transition : RateTransition  Deterministic=off  OutPortSampleTime=dt3D
  Scale : Subsystem
  Simulation 3D Scene Configuration : sim3dlib/Simulation 3D Scene Configuration  Priority=0  ProjectFormat=Default Scenes  SceneDesc=Open surface  ProjectName=C:\Program Files\MATLAB\R2021a\toolbox\shared\sim3d_projects\automotive_project\UE4\WindowsNoEditor\VehicleSimulation.exe  ScenePath=/Game/Maps/HwStrght  vehTagList={'Scene Origin'}  vehTag=Scene Origin  OpVisEn=off  Ts=dt3D  EnableWindow=on  EnableWeather=off  SunAltitude=40.0  SunAzimuth=90  clouds=10  wind=1  fog=0  rain=0  sensorTag=MainCamera1  sensorId=1  sensorName=MainCamera1  mountLoc=Origin  offsetFlag=off  tmountOffset=[0, 0, 0]  rmountOffset=[0, 0, 0]  HorizontalResolution=1280  VerticalResolution=720  HorizontalFOV=60  mountPoint=[0 0 0]  mountOrientation=[0 0 0]  aMode=aMode  ID=1
      settings: SourceProductBaseCode=DR,UV,VE
  Simulation 3D Vehicle : sim3dautolib/Simulation 3D Vehicle  Priority=-1  PassVehMesh=Muscle car  MeshPath=/MathWorksSimulation/Vehicles/Muscle/Meshes/SK_MuscleCar.SK_MuscleCar  VehColor=Red  ActorName=SimulinkVehicle1  VehLightsControl=off  HeadlightColor=[ 1, 1, 1 ]  HighBeamIntensity=100000  LowBeamIntensity=60000  HighBeamConeAngle=1.22  LowBeamConeAngle=1.22  LeftHeadlightOrientation=[ 0, 0 ]  RightHeadlightOrientation=[ 0, 0 ]  BrakelightIntensity=500  ReverselightIntensity=500  SignallightIntensity=500  SignallightPeriod=1  SignalPulseWidth=50  Translation=[VEH.InitialLongPosition VEH.InitialLatPosition -VEH.InitialVertPosition; 0 0 0; 0 0 0; 0 0 0; 0 0 0]  Rotation=[VEH.InitialRollAngle VEH.InitialPitchAngle VEH.InitialYawAngle; 0 0 0; 0 0 0; 0 0 0; 0 0 0]  Scale=ones( 5, 3 )  SampleTime=dt3D  ActorType=SimulinkVehicle  ID=1  aMode=2  ActorTag=SimulinkVehicle1
      settings: SourceProductBaseCode=DR,UV,VE
  Unary Minus : UnaryMinus
  Unary Minus1 : UnaryMinus
  wires:
  Unary Minus/1 -> Integrator/1
  Bus Selector2/1 -> Unary Minus1/1  "<dZWheel>"
  Rate Transition/1 -> Bus Selector/1, Bus Selector2/1
  Scale/1(ScaleOut) -> Simulation 3D Vehicle/3
  Demux/4 -> Part Rotation Concatenation/7(WheelRearRight Ptich)
  Demux/3 -> Part Rotation Concatenation/6(WheelRearLeft Pitch)
  Demux/2 -> Part Rotation Concatenation/5(WheelFrontRight Pitch)
  Demux/1 -> Part Rotation Concatenation/4(WheelFrontLeft Pitch)
  Constant1/1 -> Demux2/1
  Bus Selector/4 -> Data Type Conversion7/1  "<phi>"
  Part Rotation Concatenation/1(ConcatOut) -> Simulation 3D Vehicle/2
  Part Translation Concatenation/1(ConcatOut) -> Simulation 3D Vehicle/1
  Data Type Conversion12/1 -> Demux3/1
  Demux3/4 -> Part Translation Concatenation/15(WheelRearRightZ)
  Demux3/3 -> Part Translation Concatenation/14(WheelRearLeftZ)
  Demux3/1 -> Part Translation Concatenation/12(WheelFrontLeftZ)
  Demux3/2 -> Part Translation Concatenation/13(WheelFrontRightZ)
  VehFdbk/1 -> Rate Transition/1
  Data Type Conversion6/1 -> Part Translation Concatenation/3(BodyZ)
  Demux1/4 -> Part Rotation Concatenation/15(WheelRearRight Yaw)
  Demux1/3 -> Part Rotation Concatenation/14(WheelRearLeft Yaw)
  Demux2/1 -> Part Rotation Concatenation/8(WheelFrontLeft Roll)
  Demux2/2 -> Part Rotation Concatenation/9(WheelFrontRight Roll)
  Demux2/3 -> Part Rotation Concatenation/10(WheelRearLeft Roll)
  Demux2/4 -> Part Rotation Concatenation/11(WheelRearRight Roll)
  Bus Selector2/3 -> Data Type Conversion9/1  "<WhlAng>"
  Bus Selector2/2 -> Unary Minus/1  "<Omega>"
  Data Type Conversion9/1 -> Demux1/1
  Demux1/1 -> Part Rotation Concatenation/12(WheelFrontLeft Yaw)
  Demux1/2 -> Part Rotation Concatenation/13(WheelFrontRight Yaw)
  Integrator/1 -> Data Type Conversion1/1
  Data Type Conversion1/1 -> Demux/1
  Data Type Conversion8/1 -> Part Rotation Concatenation/2(Body Ptich)
  Data Type Conversion5/1 -> Part Translation Concatenation/2(BodyY)
  Data Type Conversion10/1 -> Part Rotation Concatenation/3(Body Yaw)
  Constant2/1 -> Part Translation Concatenation/5(WheelFrontRightX), Part Translation Concatenation/6(WheelRearLeftX), Part Translation Concatenation/7(WheelRearRightX), Part Translation Concatenation/8(WheelFrontLeftY), Part Translation Concatenation/9(WheelFrontRightY), Part Translation Concatenation/10(WheelRearLeftY), Part Translation Concatenation/11(WheelRearRightY), Part Translation Concatenation/4(WheelFrontLeftX)
  Data Type Conversion4/1 -> Part Translation Concatenation/1(BodyX)
  Data Type Conversion7/1 -> Part Rotation Concatenation/1(Body Roll)
  Bus Selector/1 -> Data Type Conversion4/1  "<X>"
  Bus Selector/2 -> Data Type Conversion5/1  "<Y>"
  Bus Selector/3 -> Data Type Conversion6/1  "<Z>"
  Unary Minus1/1 -> Data Type Conversion12/1
  Bus Selector/5 -> Data Type Conversion8/1  "<theta>"
  Bus Selector/6 -> Data Type Conversion10/1  "<psi>"

== system DriverInLoopSpeedgoat/3D Engine1/3D Engine Disabled ==
  VehFdbk : Inport
  Terminator : Terminator
  wires:
  VehFdbk/1 -> Terminator/1

== system DriverInLoopSpeedgoat/Controllers/Brake Controller ==
  BrkCmd : Inport
  xdot : Inport  Port=2
  kappa : Inport  Port=3
  Abs : Abs  ZeroCross=off
  Bang Bang ABS : Subsystem  VariantControl=1
  Constant1 : Constant  Value=-20
  Gain3 : Gain
  Integrator2 : Integrator  LimitOutput=on  UpperSaturationLimit=1  LowerSaturationLimit=0
  Saturation : Saturate  UpperLimit=1  LowerLimit=0  ZeroCross=off
  Switch1 : Switch  Criteria=u2 > Threshold  Threshold=.1
  Vector Concatenate2 : Concatenate  NumInputs=4
  PCmd : Outport  VectorParamsAs1DForOutWhenUnconnected=off
  wires:
  Constant1/1 -> Switch1/3
  Gain3/1 -> Switch1/1
  Saturation/1 -> Bang Bang ABS/3(<Kappa>)  "Kappa"
  Bang Bang ABS/1(PCmd) -> PCmd/1
  kappa/1 -> Abs/1
  Integrator2/1 -> Vector Concatenate2/4, Vector Concatenate2/3, Vector Concatenate2/2, Vector Concatenate2/1
  xdot/1 -> Bang Bang ABS/2(xdot)
  Abs/1 -> Saturation/1
  Vector Concatenate2/1 -> Bang Bang ABS/1(Pref)  "Reference P"
  BrkCmd/1 -> Switch1/2, Gain3/1
  Switch1/1 -> Integrator2/1

== system DriverInLoopSpeedgoat/Controllers/ECU ==
  <Accel> : Inport
  EngSpd : Inport  Port=2
  Acc to Torque Request : Gain  Gain=150
  Rev Limiter Control : Subsystem
  Signal Specification : SignalSpecification  Unit=rpm
  Unit Conversion : UnitConversion
  Trq Cmd1 : Outport  VectorParamsAs1DForOutWhenUnconnected=off
  wires:
  <Accel>/1 -> Acc to Torque Request/1
  Signal Specification/1 -> Rev Limiter Control/2(EngSpd)  "EngSpd"
  Unit Conversion/1 -> Signal Specification/1
  EngSpd/1 -> Unit Conversion/1
  Acc to Torque Request/1 -> Rev Limiter Control/1(TrqCmd)
  Rev Limiter Control/1(TrqCmdRevLimited) -> Trq Cmd1/1

== system DriverInLoopSpeedgoat/Controllers/Man_speed_control ==
  u : Inport
  Init_acc : Inport  Port=2
  Clock : Clock
  Constant : Constant  Value=stop_pedal
  From Workspace : FromWorkspace  VariableName=man_speed
  PID Controller : pid_lib/PID Controller  Controller=PID  Form=Ideal  TimeDomain=Continuous-time  UseExternalTs=off  SampleTime=-1  IntegratorMethod=Forward Euler  FilterMethod=Forward Euler  ControllerParametersSource=internal  P=1  I=0.5  D=0.02  UseFilter=on  N=100  TunerSelectOption=Transfer Function Based (PID Tuner App)  InitialConditionSource=internal  InitialConditionForIntegrator=0  InitialConditionForFilter=0  DifferentiatorICPrevScaledInput=0  ExternalReset=level  TrackingMode=off  Kt=1  LimitOutput=on  SatLimitsSource=internal  UpperSaturationLimit=1  LowerSaturationLimit=0  LinearizeAsGain=on  AntiWindupMode=clamping  Kb=1  POutMin=[]  POutMax=[]  IOutMin=[]  IOutMax=[]  DOutMin=[]  DOutMax=[]  NOutMin=[]  NOutMax=[]  SumOutMin=[]  SumOutMax=[]  SaturationOutMin=[]  SaturationOutMax=[]  PParamMin=[]  PParamMax=[]  IParamMin=[]  IParamMax=[]  DParamMin=[]  DParamMax=[]  NParamMin=[]  NParamMax=[]  KbParamMin=[]  KbParamMax=[]  KtParamMin=[]  KtParamMax=[]  KbOutMin=[]  KbOutMax=[]  KtOutMin=[]  KtOutMax=[]  IntegratorOutMin=[]  IntegratorOutMax=[]  FilterOutMin=[]  FilterOutMax=[]  SumI1OutMin=[]  SumI1OutMax=[]  SumI2OutMin=[]  SumI2OutMax=[]  SumI3OutMin=[]  SumI3OutMax=[]  SumI4OutMin=[]  SumI4OutMax=[]  SumDOutMin=[]  SumDOutMax=[]  DifferentiatorOutMin=[]  DifferentiatorOutMax=[]  FilterDiffOutCoefMin=[]  FilterDiffOutCoefMax=[]  ReciprocalOutMin=[]  ReciprocalOutMax=[]  SumDenOutMin=[]  SumDenOutMax=[]  SumNumOutMin=[]  SumNumOutMax=[]  DivideOutMin=[]  DivideOutMax=[]  UdiffTsProdOutMin=[]  UdiffTsProdOutMax=[]  NTsProdOutMin=[]  NTsProdOutMax=[]  UintegralTsProdOutMin=[]  UintegralTsProdOutMax=[]  UngainTsProdOutMin=[]  UngainTsProdOutMax=[]  IntegratorContinuousStateAttributes=''  IntegratorStateMustResolveToSignalObject=off  IntegratorRTWStateStorageClass=Auto  FilterContinuousStateAttributes=''  FilterStateMustResolveToSignalObject=off  FilterRTWStateStorageClass=Auto  ParallelPVariant=Passthrough  IdealPVariant=InternalParameters  IVariant=InternalParameters  DVariant=InternalParameters  IntegratorVariant=Continuous  SatVariant=Enabled  AWVariant=ContClampingIdeal  PCopyVariant=InternalParamsIdeal  TRVariant=Disabled  FdbkBlocksVariant=Forward  IdealPFdbkVariant=Disabled  SatFdbkVariant=Disabled  DerivativeFilterVariant=ContFilter  NVariant=InternalParameters  NCopyVariant=Disabled  FilterICVariant=InternalICsFilter  IntegratorICVariant=InternalICs  ExternalResetVariant=ExternalReset  TRSumVariant=Passthrough  SumFdbkVariant=Disabled  SumVariant=Sum_PID  TsampFilterVariant=InternalTs  TsampNgainVariant=Passthrough  TsampIntegralVariant=Passthrough  ExternalSaturationOutDataTypeStr=Inherit: Same as second input
  Scope : Scope  NumInputPorts=3
  Sum : Sum  Inputs=|+-
  Sum1 : Sum  Inputs=|+-
  Sum2 : Sum  Inputs=++|
  Switch : Switch  Criteria=u2 > Threshold
  <Accel> : Outport
  wires:
  u/1 -> Sum/2, Switch/3
  Sum2/1 -> <Accel>/1  "actual_acc"
  From Workspace/1 -> Switch/1
  Sum/1 -> PID Controller/2, PID Controller/1, Scope/2  "check_2"
  Switch/1 -> Sum/1
  Constant/1 -> Sum1/1
  Clock/1 -> Sum1/2
  Sum1/1 -> Scope/3, Switch/2  "check_1"
  PID Controller/1 -> Sum2/2, Scope/1  "pid_acc"
  Init_acc/1 -> Sum2/1

== system DriverInLoopSpeedgoat/Controllers/Transmission Controller ==
  Accel : Inport
  UpReq : Inport  Port=2
  DownReq : Inport  Port=3
  ToggleMode : Inport  Port=4
  EngSpd : Inport  Port=5
  PrpSpd : Inport  Port=6
  Automatic : Subsystem  TreatAsAtomicUnit=on
  Chart : Stateflow chart  TreatAsAtomicUnit=on
  Merge : Merge  InitialOutput=0
  Paddles : Subsystem  TreatAsAtomicUnit=on
  Switch Case : SwitchCase  CaseConditions={0,1}  ShowDefaultCase=off
  Gear : Outport
  tag scope: TransmissionModeVis=global
  wires:
  Chart/1(Mode) -> [TransmissionModeVis], Switch Case/1
  Switch Case/2 -> Automatic/Action
  Switch Case/1 -> Paddles/Action
  Automatic/1(Gear) -> Merge/1
  Paddles/1(Gear) -> Merge/2
  ToggleMode/1 -> Chart/1(Toggle)
  Merge/1 -> Gear/1
  Accel/1 -> Automatic/1(Accel)
  EngSpd/1 -> Automatic/2(EngSpd)
  PrpSpd/1 -> Automatic/3(PrpSpd)
  UpReq/1 -> Paddles/1(UpReq)
  DownReq/1 -> Paddles/2(DownReq)

== system DriverInLoopSpeedgoat/Environment/Friction Scaling ==
  note: 1) Add Subsystem or Model blocks as valid variant choices.
      | 2) You cannot connect blocks at this level. At simulation, connectivity is automatically
      | determined, based on the active variant and port name matching.
  VehFdbk : Inport
  Constant : Subsystem  VariantControl=0
  Lookup Table : Subsystem  VariantControl=1
  mu : Outport  VectorParamsAs1DForOutWhenUnconnected=off

== system DriverInLoopSpeedgoat/Environment/Ground Height ==
  note: 1) Add Subsystem or Model blocks as valid variant choices.
      | 2) You cannot connect blocks at this level. At simulation, connectivity is automatically
      | determined, based on the active variant and port name matching.
  3D Engine : Subsystem  VariantControl=1
  Constant : Subsystem  VariantControl=0
  z : Outport  VectorParamsAs1DForOutWhenUnconnected=off

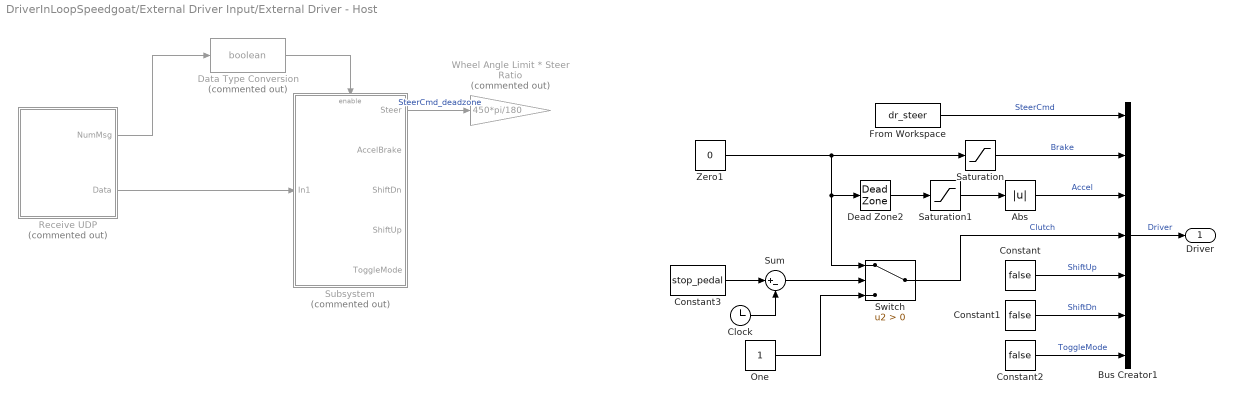
== system DriverInLoopSpeedgoat/External Driver Input/External Driver - Host ==
  Abs : Abs
  Bus Creator1 : BusCreator  Inputs=7
  Clock : Clock
  Constant : Constant  Value=false
  Constant1 : Constant  Value=false
  Constant2 : Constant  Value=false
  Constant3 : Constant  Value=stop_pedal
  Data Type Conversion : DataTypeConversion  Commented=on  OutDataTypeStr=boolean
  Dead Zone2 : DeadZone  LowerValue=-0.0078  UpperValue=0
  From Workspace : FromWorkspace  VariableName=dr_steer
  One : Constant  OutDataTypeStr=Inherit: Inherit via back propagation
  Receive UDP : Subsystem  Commented=on  TreatAsAtomicUnit=on
  Saturation : Saturate  UpperLimit=1  LowerLimit=0
  Saturation1 : Saturate  UpperLimit=0  LowerLimit=-1
  Subsystem : Subsystem  Commented=on
  Sum : Sum  Inputs=|+-
  Switch : Switch  Criteria=u2 > Threshold
  Wheel Angle Limit * Steer Ratio : Gain  Commented=on  Gain=450*pi/180
  Zero1 : Constant  Value=0  OutDataTypeStr=Inherit: Inherit via back propagation
  Driver : Outport  VectorParamsAs1DForOutWhenUnconnected=off
  wires:
  Saturation/1 -> Bus Creator1/2  "Brake"
  Saturation1/1 -> Abs/1
  Subsystem/1(Steer) -> Wheel Angle Limit * Steer Ratio/1  "SteerCmd_deadzone"
  Switch/1 -> Bus Creator1/4  "Clutch"
  Bus Creator1/1 -> Driver/1  "Driver"
  Dead Zone2/1 -> Saturation1/1
  Abs/1 -> Bus Creator1/3  "Accel"
  Receive UDP/2(Data) -> Subsystem/1(In1)
  Data Type Conversion/1 -> Subsystem/Enable
  Receive UDP/1(NumMsg) -> Data Type Conversion/1
  Constant1/1 -> Bus Creator1/6  "ShiftDn"
  From Workspace/1 -> Bus Creator1/1  "SteerCmd"
  Constant2/1 -> Bus Creator1/7  "ToggleMode"
  Constant/1 -> Bus Creator1/5  "ShiftUp"
  Zero1/1 -> Switch/1, Dead Zone2/1, Saturation/1
  One/1 -> Switch/3
  Sum/1 -> Switch/2
  Clock/1 -> Sum/2
  Constant3/1 -> Sum/1

== system DriverInLoopSpeedgoat/External Driver Input/External Driver - Speedgoat ==
  Bus Creator : BusCreator  Inputs=2
  Bus Creator1 : BusCreator  Inputs=5
  Data Type Conversion : DataTypeConversion  OutDataTypeStr=double
  Data Type Conversion1 : DataTypeConversion  OutDataTypeStr=double
  MapAndScaleAxes : Subsystem  VariantControl=LogitechG920
  MapButtons : Subsystem  VariantControl=LogitechG920
  Mux : Mux  Inputs=2
  "Steering Wheel Read " : slrealtimeobsoletelib/Obsolete  ObsoleteBlock=logitechG29/Steering Wheel Read  ObsoleteParameters="MultiThreadCoSim:  auto sampleTime:  1e-3"  NumInports=0  NumOutports=5
      settings: SourceProductName=Simulink Real-Time
  Terminator : Terminator
  Terminator1 : Terminator
  Terminator2 : Terminator
  Driver : Outport  VectorParamsAs1DForOutWhenUnconnected=off
  wires:
  MapAndScaleAxes/4(Clutch) -> Bus Creator1/4  "Clutch"
  Bus Creator/1 -> Bus Creator1/5  "ShiftCmd"
  Bus Creator1/1 -> Driver/1
  MapAndScaleAxes/3(Brake) -> Bus Creator1/3  "Brake"
  MapAndScaleAxes/2(Accel) -> Bus Creator1/2  "Accel"
  MapAndScaleAxes/1(Steering) -> Bus Creator1/1  "Steer"
  "Steering Wheel Read "/4 -> Terminator/1
  "Steering Wheel Read "/5 -> Terminator1/1
  Mux/1 -> MapAndScaleAxes/1(WheelPedals)  "SteeringWheelAxes"
  "Steering Wheel Read "/3 -> Data Type Conversion1/1
  Data Type Conversion1/1 -> Mux/2
  "Steering Wheel Read "/2 -> Data Type Conversion/1
  Data Type Conversion/1 -> Mux/1
  "Steering Wheel Read "/1 -> MapButtons/1(Buttons)  "SteeringWheelButtons"
  MapButtons/1(LeftPaddle) -> Bus Creator/1  "ShiftDn"
  MapButtons/2(RightPaddle) -> Bus Creator/2  "ShiftUp"
  MapButtons/3(AllButtons) -> Terminator2/1

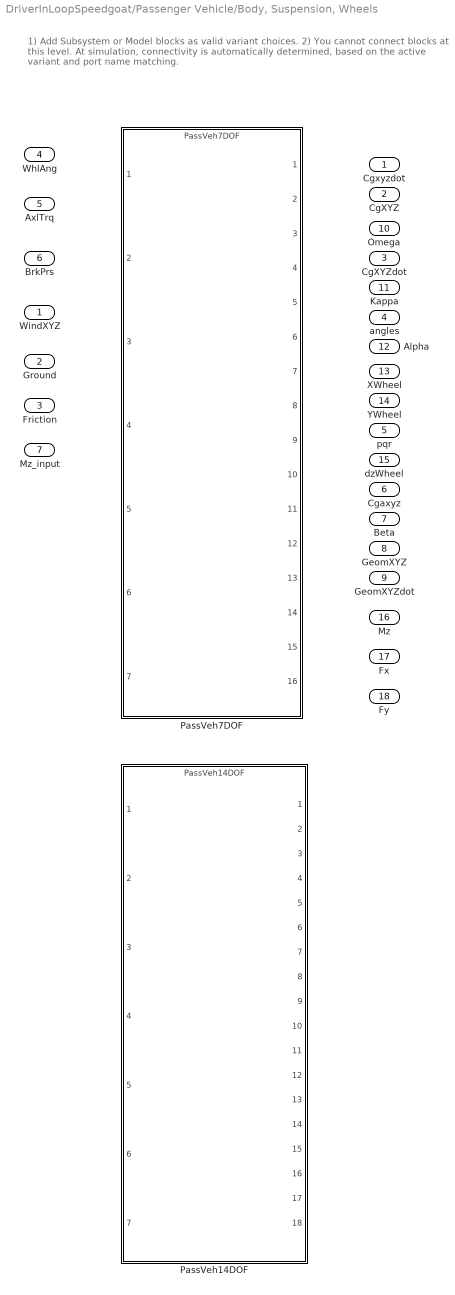
== system DriverInLoopSpeedgoat/Passenger Vehicle/Body, Suspension, Wheels ==
  note: 1) Add Subsystem or Model blocks as valid variant choices.
      | 2) You cannot connect blocks at this level. At simulation, connectivity is automatically
      | determined, based on the active variant and port name matching.
  WindXYZ : Inport
  Ground : Inport  Port=2  PortDimensions=4
  Friction : Inport  Port=3  PortDimensions=4
  WhlAng : Inport  Port=4
  AxlTrq : Inport  Port=5
  BrkPrs : Inport  Port=6
  Mz_input : Inport  Port=7
  PassVeh14DOF : ModelReference  DisableCoverage=on  ModelNameDialog=PassVeh14DOF  SimulationMode=Normal  VariantControl=3  ModelReferenceVersion=3.9
  PassVeh7DOF : ModelReference  DisableCoverage=on  ModelNameDialog=PassVeh7DOF  SimulationMode=Normal  VariantControl=1  ModelReferenceVersion=2.0
  Cgxyzdot : Outport  VectorParamsAs1DForOutWhenUnconnected=off
  CgXYZ : Outport  Port=2  VectorParamsAs1DForOutWhenUnconnected=off
  CgXYZdot : Outport  Port=3  VectorParamsAs1DForOutWhenUnconnected=off
  angles : Outport  Port=4  VectorParamsAs1DForOutWhenUnconnected=off
  pqr : Outport  Port=5  VectorParamsAs1DForOutWhenUnconnected=off
  Cgaxyz : Outport  Port=6  VectorParamsAs1DForOutWhenUnconnected=off
  Beta : Outport  Port=7  VectorParamsAs1DForOutWhenUnconnected=off
  GeomXYZ : Outport  Port=8  VectorParamsAs1DForOutWhenUnconnected=off
  GeomXYZdot : Outport  Port=9  VectorParamsAs1DForOutWhenUnconnected=off
  Omega : Outport  Port=10  PortDimensions=4  VectorParamsAs1DForOutWhenUnconnected=off
  Kappa : Outport  Port=11  PortDimensions=4  VectorParamsAs1DForOutWhenUnconnected=off
  Alpha : Outport  Port=12  PortDimensions=4  VectorParamsAs1DForOutWhenUnconnected=off
  XWheel : Outport  Port=13  VectorParamsAs1DForOutWhenUnconnected=off
  YWheel : Outport  Port=14  VectorParamsAs1DForOutWhenUnconnected=off
  dzWheel : Outport  Port=15  VectorParamsAs1DForOutWhenUnconnected=off
  Mz : Outport  Port=16  VectorParamsAs1DForOutWhenUnconnected=off
  Fx : Outport  Port=17  VectorParamsAs1DForOutWhenUnconnected=off
  Fy : Outport  Port=18  VectorParamsAs1DForOutWhenUnconnected=off

== system DriverInLoopSpeedgoat/Passenger Vehicle/Clutch_action ==
  "EngTrq " : Inport
  Operator : Inport  Port=2
  Bus Creator : BusCreator  Inputs=1
  Bus Selector : BusSelector  OutputSignals=Clutch
  Clutch_scaled_torque : Product  Inputs=**
  One : Constant  OutDataTypeStr=Inherit: Inherit via back propagation
  Sum : Sum  Inputs=-+|
  Eng : Outport  VectorParamsAs1DForOutWhenUnconnected=off
  wires:
  "EngTrq "/1 -> Clutch_scaled_torque/2
  Bus Creator/1 -> Eng/1
  Clutch_scaled_torque/1 -> Bus Creator/1  "EngTrq"
  Operator/1 -> Bus Selector/1
  Bus Selector/1 -> Sum/1  "<Clutch>"
  Sum/1 -> Clutch_scaled_torque/1
  One/1 -> Sum/2

== system DriverInLoopSpeedgoat/Passenger Vehicle/Engine ==
  note: 1) Add Subsystem or Model blocks as valid variant choices.
      | 2) You cannot connect blocks at this level. At simulation, connectivity is automatically
      | determined, based on the active variant and port name matching.
  TrqCmd : Inport
  EngSpd : Inport  Port=2  Unit=rad/s
  Ideal Mapped Engine : ModelReference  DisableCoverage=on  ModelNameDialog=SiMappedEngineV  SimulationMode=Normal  VariantControl=0  ModelReferenceVersion=3.2
  EngTrq : Outport  VectorParamsAs1DForOutWhenUnconnected=off

== system DriverInLoopSpeedgoat/Passenger Vehicle/Steering, Transmission, Driveline and Brakes ==
  note: 1) Add Subsystem or Model blocks as valid variant choices.
      | 2) You cannot connect blocks at this level. At simulation, connectivity is automatically
      | determined, based on the active variant and port name matching.
  SteerHWCmd : Inport
  EngTrq : Inport  Port=2
  GearCmd : Inport  Port=3  OutDataTypeStr=int8
  BrkPrsCmd : Inport  Port=4  PortDimensions=4
  Omega : Inport  Port=5
  Driveline Ideal Fixed Gear : ModelReference  DisableCoverage=on  ModelNameDialog=Driveline  SimulationMode=Normal  VariantControl=0  ModelReferenceVersion=3.1
  WhlAng : Outport  VectorParamsAs1DForOutWhenUnconnected=off
  AxlTrq : Outport  Port=2  VectorParamsAs1DForOutWhenUnconnected=off
  BrkPrs : Outport  Port=3  PortDimensions=4  VectorParamsAs1DForOutWhenUnconnected=off
  EngSpd : Outport  Port=4  Unit=rad/s  VectorParamsAs1DForOutWhenUnconnected=off
  PropShftSpd : Outport  Port=5  VectorParamsAs1DForOutWhenUnconnected=off

== system DriverInLoopSpeedgoat/Passenger Vehicle/Subsystem ==
  Env : Inport
  Driveline : Inport  Port=2
  Bus Selector1 : BusSelector  OutputSignals=Gnd.signal1.z.G_FL_z,Gnd.signal1.z.G_FR_z,Gnd.signal1.z.G_RL_z,Gnd.signal1.z.G_RR_z
  Bus Selector2 : BusSelector  OutputSignals=Wind
  Bus Selector3 : BusSelector  OutputSignals=Gnd.mu.mu_FL,Gnd.mu.mu_FR,Gnd.mu.mu_RL,Gnd.mu.mu_RR
  Bus Selector4 : BusSelector  OutputSignals=WhlAng,AxlTrq,BrkPrs
  Vector Concatenate : Concatenate  NumInputs=4
  Vector Concatenate1 : Concatenate  NumInputs=4
  Wind : Outport  VectorParamsAs1DForOutWhenUnconnected=off
  Gnd : Outport  Port=2  VectorParamsAs1DForOutWhenUnconnected=off
  mu : Outport  Port=3  VectorParamsAs1DForOutWhenUnconnected=off
  WhlAng : Outport  Port=4  VectorParamsAs1DForOutWhenUnconnected=off
  AxlTrq : Outport  Port=5  VectorParamsAs1DForOutWhenUnconnected=off
  BrkPrs : Outport  Port=6  VectorParamsAs1DForOutWhenUnconnected=off
  wires:
  Env/1 -> Bus Selector3/1, Bus Selector1/1, Bus Selector2/1
  Bus Selector2/1 -> Wind/1  "<Wind>"
  Bus Selector3/1 -> Vector Concatenate/1  "<mu_FL>"
  Bus Selector3/2 -> Vector Concatenate/2  "<mu_FR>"
  Bus Selector3/3 -> Vector Concatenate/3  "<mu_RL>"
  Bus Selector3/4 -> Vector Concatenate/4  "<mu_RR>"
  Vector Concatenate/1 -> mu/1
  Bus Selector1/1 -> Vector Concatenate1/1  "<G_FL_z>"
  Bus Selector1/2 -> Vector Concatenate1/2  "<G_FR_z>"
  Bus Selector1/3 -> Vector Concatenate1/3  "<G_RL_z>"
  Bus Selector1/4 -> Vector Concatenate1/4  "<G_RR_z>"
  Vector Concatenate1/1 -> Gnd/1
  Driveline/1 -> Bus Selector4/1
  Bus Selector4/2 -> AxlTrq/1  "<AxlTrq>"
  Bus Selector4/1 -> WhlAng/1  "<WhlAng>"
  Bus Selector4/3 -> BrkPrs/1  "<BrkPrs>"

== system DriverInLoopSpeedgoat/Passenger Vehicle/Subsystem1 ==
  WhlAng : Inport
  AxlTrq : Inport  Port=2
  BrkPrs : Inport  Port=3
  EngSpd : Inport  Port=4
  PropShftSpd : Inport  Port=5
  Bus Creator1 : BusCreator  Inputs=5
  Driveline : Outport  VectorParamsAs1DForOutWhenUnconnected=off
  wires:
  Bus Creator1/1 -> Driveline/1  "Driveline"
  PropShftSpd/1 -> Bus Creator1/5  "PropShftSpd"
  AxlTrq/1 -> Bus Creator1/2  "AxlTrq"
  WhlAng/1 -> Bus Creator1/1  "WhlAng"
  EngSpd/1 -> Bus Creator1/4  "EngSpd"
  BrkPrs/1 -> Bus Creator1/3  "BrkPrs"

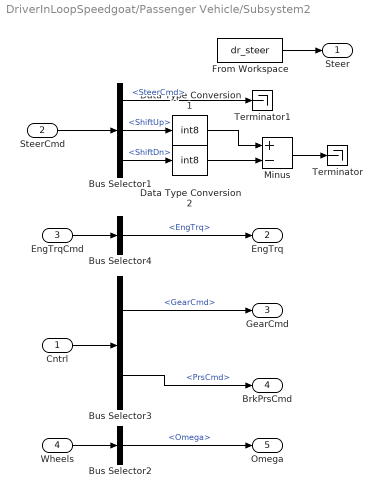
== system DriverInLoopSpeedgoat/Passenger Vehicle/Subsystem2 ==
  Cntrl : Inport
  SteerCmd : Inport  Port=2
  EngTrqCmd : Inport  Port=3
  Wheels : Inport  Port=4
  Bus Selector1 : BusSelector  OutputSignals=SteerCmd,ShiftUp,ShiftDn
  Bus Selector2 : BusSelector  OutputSignals=Omega
  Bus Selector3 : BusSelector  OutputSignals=Transmission.GearCmd,Brake.PrsCmd
  Bus Selector4 : BusSelector  OutputSignals=EngTrq
  Data Type Conversion1 : DataTypeConversion  OutDataTypeStr=int8
  Data Type Conversion2 : DataTypeConversion  OutDataTypeStr=int8
  From Workspace : FromWorkspace  VariableName=dr_steer
  Minus : Sum  Inputs=+-
  Terminator : Terminator
  Terminator1 : Terminator
  Steer : Outport  VectorParamsAs1DForOutWhenUnconnected=off
  EngTrq : Outport  Port=2  VectorParamsAs1DForOutWhenUnconnected=off
  GearCmd : Outport  Port=3  VectorParamsAs1DForOutWhenUnconnected=off
  BrkPrsCmd : Outport  Port=4  VectorParamsAs1DForOutWhenUnconnected=off
  Omega : Outport  Port=5  VectorParamsAs1DForOutWhenUnconnected=off
  wires:
  Cntrl/1 -> Bus Selector3/1
  Bus Selector3/1 -> GearCmd/1  "<GearCmd>"
  SteerCmd/1 -> Bus Selector1/1
  Wheels/1 -> Bus Selector2/1
  Bus Selector2/1 -> Omega/1  "<Omega>"
  Bus Selector3/2 -> BrkPrsCmd/1  "<PrsCmd>"
  EngTrqCmd/1 -> Bus Selector4/1
  Bus Selector1/1 -> Terminator1/1  "<SteerCmd>"
  Bus Selector4/1 -> EngTrq/1  "<EngTrq>"
  Minus/1 -> Terminator/1
  Bus Selector1/2 -> Data Type Conversion1/1  "<ShiftUp>"
  Bus Selector1/3 -> Data Type Conversion2/1  "<ShiftDn>"
  Data Type Conversion1/1 -> Minus/1
  Data Type Conversion2/1 -> Minus/2
  From Workspace/1 -> Steer/1

== system DriverInLoopSpeedgoat/Passenger Vehicle/Subsystem3 ==
  Cntrl : Inport
  Driveline : Inport  Port=2
  Bus Selector : BusSelector  OutputSignals=ECU.EngTrqCmd
  Bus Selector1 : BusSelector  OutputSignals=EngSpd
  EngTrqCmd : Outport  VectorParamsAs1DForOutWhenUnconnected=off
  EngSpd : Outport  Port=2  VectorParamsAs1DForOutWhenUnconnected=off
  wires:
  Driveline/1 -> Bus Selector1/1
  Cntrl/1 -> Bus Selector/1
  Bus Selector/1 -> EngTrqCmd/1  "<EngTrqCmd>"
  Bus Selector1/1 -> EngSpd/1  "<EngSpd>"
